simulink subsystem "MacPhersonSuspensionFront"  (R2024b)
settings: Solver=VariableStepAuto  StartTime=0.0  StopTime=10.0  RelTol=1e-3
undefined symbols (not defined in the file): PlntVehCGHgtAxl, PlntWhlNumFrnt
libraries: autolibsharedcommon x4, autolibutils x2, sharedtransform x2, matrix_library x2, vehdynlibsuspension x1
settings Model: ModifiedByFormat=The MathWorks, Inc.  Creator=The MathWorks, Inc.  LastModifiedBy=The MathWorks, Inc.
settings OptimizationCC: ReuseModelBlockBuffer=off
settings DebuggingCC: SubsystemReferenceDiagnosticForUnitTest=warning
settings RTWCC: GPUComputeCapability=3.5

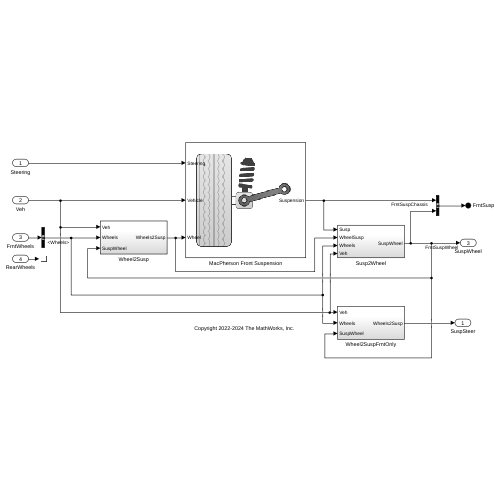
[thumbnail: Simulink's stored preview of the top-level diagram]
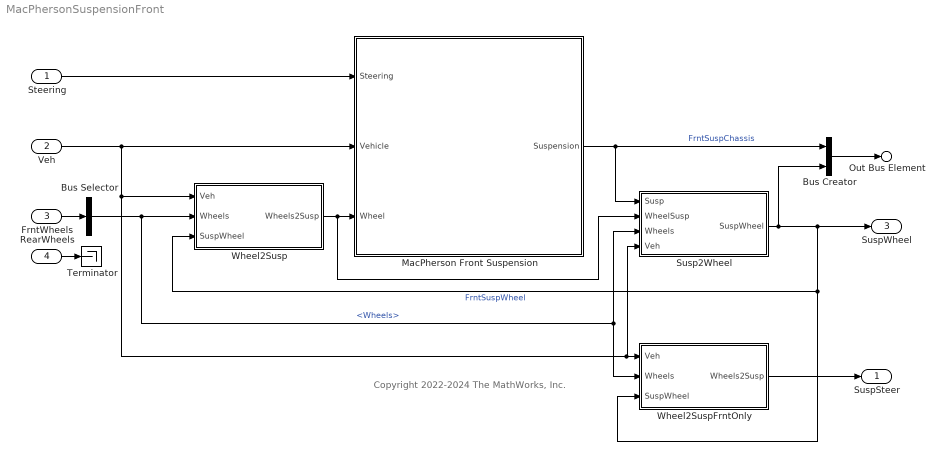
== system MacPhersonSuspensionFront ==
  note: Copyright 2022-2024 The MathWorks, Inc.
  Steering : Inport
  Veh : Inport  Port=2
  FrntWheels : Inport  Port=3
  RearWheels : Inport  Port=4
  Bus Creator : BusCreator  Inputs=2
  Bus Selector : BusSelector  OutputSignals=Wheels
  MacPherson Front Suspension : Subsystem  VariantControl=MacPherson Front Suspension Solid Axle Rear Suspension
      mask Display: image([imread('suspmacp.png')]);
  Susp2Wheel : Subsystem
  Terminator : Terminator
  Wheel2Susp : Subsystem
  Wheel2SuspFrntOnly : Subsystem
  SuspSteer : Outport
  Out Bus Element : Outport  Port=2  PortName=FrntSusp
  SuspWheel : Outport  Port=3
  wires:
  Veh/1 -> MacPherson Front Suspension/2(Vehicle), Susp2Wheel/4(Veh), Wheel2SuspFrntOnly/1(Veh), Wheel2Susp/1(Veh)
  Susp2Wheel/1(SuspWheel) -> Bus Creator/2, Wheel2SuspFrntOnly/3(SuspWheel), Wheel2Susp/3(SuspWheel), SuspWheel/1  "FrntSuspWheel"
  MacPherson Front Suspension/1(Suspension) -> Susp2Wheel/1(Susp), Bus Creator/1  "FrntSuspChassis"
  Wheel2Susp/1(Wheels2Susp) -> MacPherson Front Suspension/3(Wheel), Susp2Wheel/2(WheelSusp)
  Steering/1 -> MacPherson Front Suspension/1(Steering)
  Bus Selector/1 -> Susp2Wheel/3(Wheels), Wheel2SuspFrntOnly/2(Wheels), Wheel2Susp/2(Wheels)  "<Wheels>"
  RearWheels/1 -> Terminator/1
  FrntWheels/1 -> Bus Selector/1
  Bus Creator/1 -> Out Bus Element/1
  Wheel2SuspFrntOnly/1(Wheels2Susp) -> SuspSteer/1

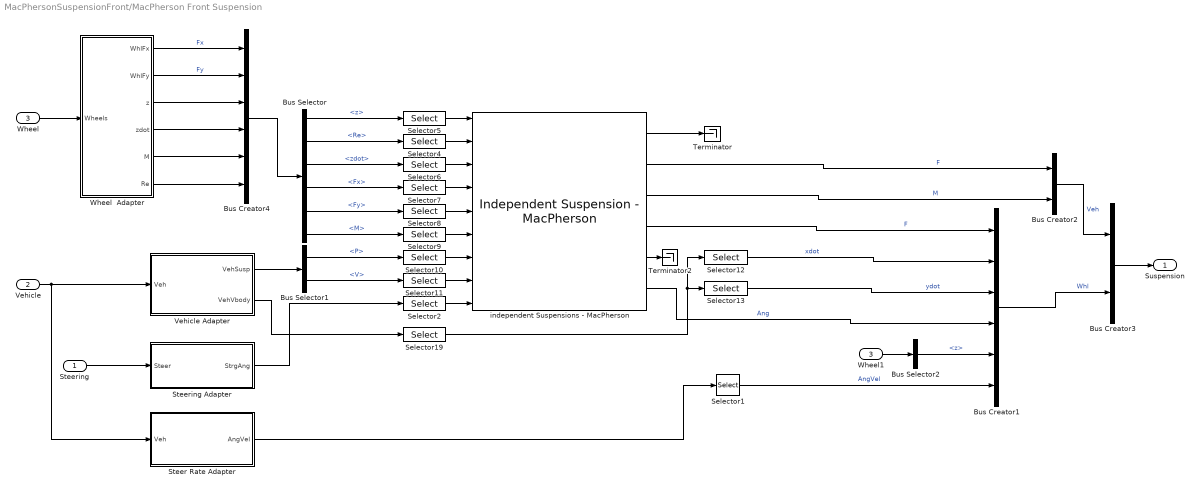
== system MacPhersonSuspensionFront/MacPherson Front Suspension ==
  Steering : Inport
  Vehicle : Inport  Port=2
  Wheel : Inport  Port=3
  Bus Creator1 : BusCreator  Inputs=6
  Bus Creator2 : BusCreator  Inputs=2
  Bus Creator3 : BusCreator  Inputs=2
  Bus Creator4 : BusCreator  Inputs=6
  Bus Selector : BusSelector  OutputSignals=z,Re,zdot,Fx,Fy,M
  Bus Selector1 : BusSelector  OutputSignals=P,V
  Bus Selector2 : BusSelector  OutputSignals=SuspFrame.z
  Selector1 : Selector  NumberOfDimensions=2  InputPortWidth=4  IndexOptions=Index vector (dialog),Index vector (dialog)  Indices=[1 2 3],[1 2]  OutputSizes=1,1
  Selector{9..11,19} (4 alike) : Selector  NumberOfDimensions=2  IndexOptions=Select all,Index vector (dialog)  Indices=[1 2],[1 2]  OutputSizes=1,1
  Selector12 : Selector  NumberOfDimensions=2  InputPortWidth=3  IndexOptions=Index vector (dialog),Select all  Indices=1,1  OutputSizes=1,1
  Selector13 : Selector  NumberOfDimensions=2  InputPortWidth=3  IndexOptions=Index vector (dialog),Select all  Indices=2,1  OutputSizes=1,1
  Selector{2,4..8} (6 alike) : Selector  IndexOptions=Index vector (dialog)  Indices=[1 2]  OutputSizes=1
  Steer Rate Adapter : Subsystem
  Steering Adapter : Subsystem
  Terminator : Terminator
  Terminator2 : Terminator
  Vehicle Adapter : Subsystem
  Wheel  Adapter : Subsystem
  Wheel1 : InportShadow  Port=3
  independent Suspensions - MacPherson : vehdynlibsuspension/Independent Suspension - MacPherson  ActiveDampEn=off  NumAxl=1  NumWhlsByAxl=2  StrgEnByAxl=1  AntiSwayEnByAxl=1  WhlNumVec="[1  2]"  AxleNumVec="[1  1]"  SuspTypesByAxle=[1]  SuspImage=suspmacp.png  IdealSuspEn=on  IdealSuspAxles=[1]  Kz=PlntSpMSStiffness  F0z=PlntSpMSPreload  Cz=PlntSpMSDamping  Hmax=PlntSpMSMaxHeight  f_act_susp_cz=[10000 10000;10000 10000]  f_act_susp_duty_bpt=[0 1]  f_act_susp_zdot_bpt=[-1 1]  Toe=PlntSpMSStatToe  RollStrgSlp=0.  ToeStrgSlp=0.  Caster=PlntSpMSStatCaster  CasterHslp=0.  CasterStrgSlp=0.  Camber=PlntSpMSStatCamber  CamberHslp=0.  CamberStrgSlp=0.  StrgHgtSlp=PlntSpMSHeightVsSteer  MappedSuspEn=off  MappedSuspAxles="[1  2]"  f_susp_axl_bp=[1 2]  f_susp_dz_bp=[-0.15 -0.14 -0.13 -0.12 -0.11 -0.10 -0.09 -0.08 -0.07 -0.06 -0.05 -0.04 -0.03 -0.02 -0.01 0.00 0.01 0.02 0.03 0.04 0.05 0.06 0.07 0.08 0.09 0.10 0.11 0.12 0.13 0.14 0.15]  f_susp_dzdot_bp=[-0.15 -0.14 -0.13 -0.12 -0.11 -0.10 -0.09 -0.08 -0.07 -0.06 -0.05 -0.04 -0.03 -0.02 -0.01 0.00 0.01 0.02 0.03 0.04 0.05 0.06 0.07 0.08 0.09 0.10 0.11 0.12 0.13 0.14 0.15]  f_susp_fmz=zeros(31,31,61,2,4)  f_susp_geom=zeros(31,61,2,3)  f_susp_strgdelta_bp=[-30,-29,-28,-27,-26,-25,-24,-23,-22,-21,-20,-19,-18,-17,-16,-15,-14,-13,-12,-11,-10,-9,-8,-7,-6,-5,-4,-3,-2,-1,0,1,2,3,4,5,6,7,8,9,10,11,12,13,14,15,16,17,18,19,20,21,22,23,24,25,26,27,28,29,30]  AntiSwayR=PlntSpMSAntiSwayRadius  AntiSwayNtrlAng=PlntSpMSAntiSwayNeutralAngle  AntiSwayTrsK=PlntSpMSAntiSwayTorsionStiffness
  Suspension : Outport  VectorParamsAs1DForOutWhenUnconnected=off
  wires:
  Selector1/1 -> Bus Creator1/6  "AngVel"
  Bus Selector2/1 -> Bus Creator1/5  "<z>"
  Wheel1/1 -> Bus Selector2/1
  Selector19/1 -> Selector13/1, Selector12/1
  independent Suspensions - MacPherson/5 -> Terminator2/1
  Steer Rate Adapter/1(AngVel) -> Selector1/1
  Vehicle Adapter/2(VehVbody) -> Selector19/1
  Bus Selector/3 -> Selector6/1  "<zdot>"
  Vehicle/1 -> Steer Rate Adapter/1(Veh), Vehicle Adapter/1(Veh)
  Wheel  Adapter/6(Re) -> Bus Creator4/6
  independent Suspensions - MacPherson/2 -> Bus Creator2/1  "F"
  independent Suspensions - MacPherson/3 -> Bus Creator2/2  "M"
  independent Suspensions - MacPherson/4 -> Bus Creator1/1  "F"
  independent Suspensions - MacPherson/6 -> Bus Creator1/4  "Ang"
  Selector12/1 -> Bus Creator1/2  "xdot"
  Selector11/1 -> independent Suspensions - MacPherson/8
  Selector10/1 -> independent Suspensions - MacPherson/7
  Selector9/1 -> independent Suspensions - MacPherson/6
  Selector8/1 -> independent Suspensions - MacPherson/5
  Selector7/1 -> independent Suspensions - MacPherson/4
  Selector6/1 -> independent Suspensions - MacPherson/3
  Selector5/1 -> independent Suspensions - MacPherson/1
  Selector4/1 -> independent Suspensions - MacPherson/2
  Selector2/1 -> independent Suspensions - MacPherson/9
  Bus Selector/2 -> Selector4/1  "<Re>"
  Wheel  Adapter/5(M) -> Bus Creator4/5
  Wheel  Adapter/4(zdot) -> Bus Creator4/4
  Wheel  Adapter/3(z) -> Bus Creator4/3
  Wheel/1 -> Wheel  Adapter/1(Wheels)
  Wheel  Adapter/1(WhlFx) -> Bus Creator4/1  "Fx"
  Wheel  Adapter/2(WhlFy) -> Bus Creator4/2  "Fy"
  Bus Creator4/1 -> Bus Selector/1
  Steering Adapter/1(StrgAng) -> Selector2/1
  Bus Creator2/1 -> Bus Creator3/1  "Veh"
  Vehicle Adapter/1(VehSusp) -> Bus Selector1/1
  Bus Selector/4 -> Selector7/1  "<Fx>"
  independent Suspensions - MacPherson/1 -> Terminator/1
  Selector13/1 -> Bus Creator1/3  "ydot"
  Bus Selector1/1 -> Selector10/1  "<P>"
  Steering/1 -> Steering Adapter/1(Steer)
  Bus Selector/1 -> Selector5/1  "<z>"
  Bus Selector/5 -> Selector8/1  "<Fy>"
  Bus Selector/6 -> Selector9/1  "<M>"
  Bus Selector1/2 -> Selector11/1  "<V>"
  Bus Creator1/1 -> Bus Creator3/2  "Whl"
  Bus Creator3/1 -> Suspension/1

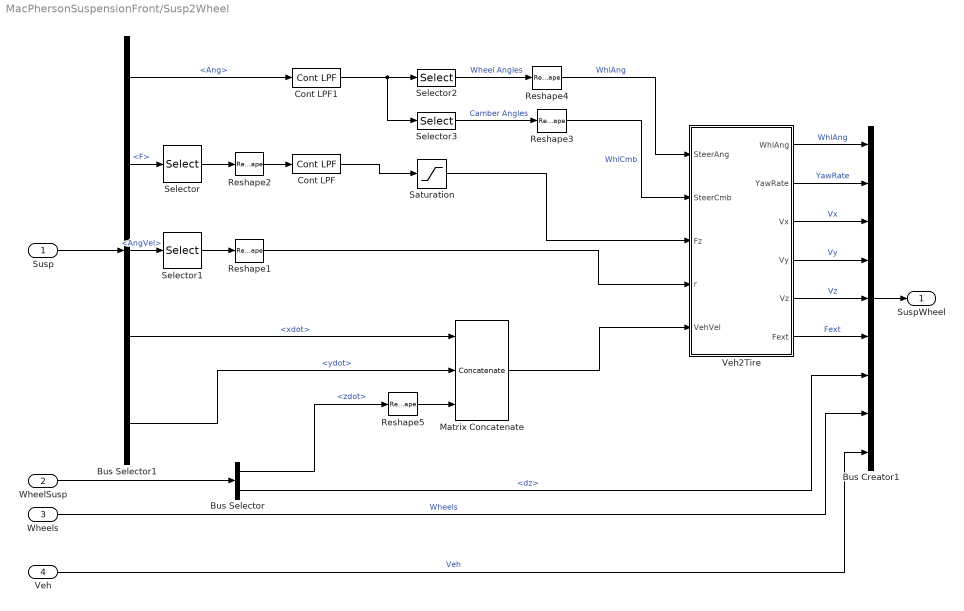
== system MacPhersonSuspensionFront/Susp2Wheel ==
  Susp : Inport
  WheelSusp : Inport  Port=2
  Wheels : Inport  Port=3
  Veh : Inport  Port=4
  Bus Creator1 : BusCreator  Inputs=9
  Bus Selector : BusSelector  OutputSignals=SuspFrame.zdot,SuspFrame.dz
  Bus Selector1 : BusSelector  OutputSignals=Whl.Ang,Whl.F,Whl.AngVel,Whl.xdot,Whl.ydot
  Cont LPF : autolibutils/Cont LPF  wc=100*2*pi  AbsoluteTolerance=auto  aMode=2
  Cont LPF1 : autolibutils/Cont LPF  wc=100*2*pi  AbsoluteTolerance=auto  aMode=2
  Matrix Concatenate : Concatenate  NumInputs=3  Mode=Multidimensional array
  Reshape{1..4} (4 alike) : Reshape
  Reshape5 : Reshape  OutputDimensionality=Row vector (2-D)
  Saturation : Saturate  UpperLimit=inf  LowerLimit=-10*9.81*2000  ZeroCross=off
  Selector : Selector  NumberOfDimensions=2  InputPortWidth=3  IndexOptions=Index vector (dialog),Select all  Indices=[3],1  OutputSizes=1,1
  Selector1 : Selector  NumberOfDimensions=2  InputPortWidth=1  IndexOptions=Index vector (dialog),Select all  Indices=[3],1  OutputSizes=1,1
  Selector2 : Selector  NumberOfDimensions=2  InputPortWidth=3  IndexOptions=Index vector (dialog),Select all  Indices=3,1  OutputSizes=1,1
  Selector3 : Selector  NumberOfDimensions=2  InputPortWidth=3  IndexOptions=Index vector (dialog),Select all  Indices=1,1  OutputSizes=1,1
  Veh2Tire : Subsystem
  SuspWheel : Outport
  wires:
  Bus Creator1/1 -> SuspWheel/1
  Bus Selector/1 -> Reshape5/1  "<zdot>"
  Veh2Tire/3(Vx) -> Bus Creator1/3  "Vx"
  Veh2Tire/4(Vy) -> Bus Creator1/4  "Vy"
  Susp/1 -> Bus Selector1/1
  Veh2Tire/5(Vz) -> Bus Creator1/5  "Vz"
  Bus Selector1/1 -> Cont LPF1/1  "<Ang>"
  Reshape5/1 -> Matrix Concatenate/3
  WheelSusp/1 -> Bus Selector/1
  Cont LPF/1 -> Saturation/1
  Selector/1 -> Reshape2/1
  Matrix Concatenate/1 -> Veh2Tire/5(VehVel)
  Saturation/1 -> Veh2Tire/3(Fz)
  Selector1/1 -> Reshape1/1
  Veh2Tire/6(Fext) -> Bus Creator1/6  "Fext"
  Bus Selector1/5 -> Matrix Concatenate/2  "<ydot>"
  Bus Selector1/3 -> Selector1/1  "<AngVel>"
  Bus Selector1/4 -> Matrix Concatenate/1  "<xdot>"
  Reshape4/1 -> Veh2Tire/1(SteerAng)  "WhlAng"
  Veh2Tire/1(WhlAng) -> Bus Creator1/1  "WhlAng"
  Reshape3/1 -> Veh2Tire/2(SteerCmb)  "WhlCmb"
  Selector3/1 -> Reshape3/1  "Camber Angles"
  Reshape2/1 -> Cont LPF/1
  Selector2/1 -> Reshape4/1  "Wheel Angles"
  Reshape1/1 -> Veh2Tire/4(r)
  Cont LPF1/1 -> Selector3/1, Selector2/1
  Bus Selector1/2 -> Selector/1  "<F>"
  Veh2Tire/2(YawRate) -> Bus Creator1/2  "YawRate"
  Bus Selector/2 -> Bus Creator1/7  "<dz>"
  Wheels/1 -> Bus Creator1/8  "Wheels"
  Veh/1 -> Bus Creator1/9  "Veh"

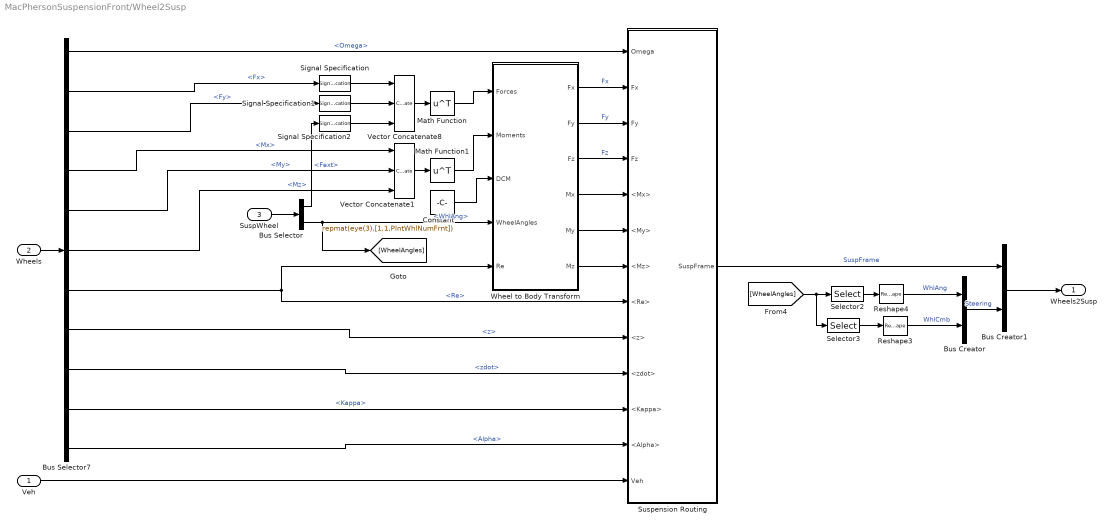
== system MacPhersonSuspensionFront/Wheel2Susp ==
  Veh : Inport
  Wheels : Inport  Port=2
  SuspWheel : Inport  Port=3
  Bus Creator : BusCreator  Inputs=2
  Bus Creator1 : BusCreator  Inputs=2
  Bus Selector : BusSelector  OutputSignals=Fext,WhlAng
  Bus Selector7 : BusSelector  OutputSignals=Omega,Fx,Fy,Mx,My,Mz,Re,z,zdot,Kappa,Alpha
  Constant : Constant  Value=repmat(eye(3),[1,1,PlntWhlNumFrnt])
  Math Function : Math  Operator=transpose  SignedPower=on
  Math Function1 : Math  Operator=transpose  SignedPower=on
  Reshape3 : Reshape
  Reshape4 : Reshape
  Selector2 : Selector  NumberOfDimensions=2  InputPortWidth=3  IndexOptions=Index vector (dialog),Select all  Indices=3,1  OutputSizes=1,1
  Selector3 : Selector  NumberOfDimensions=2  InputPortWidth=3  IndexOptions=Index vector (dialog),Select all  Indices=1,1  OutputSizes=1,1
  Signal Specification : SignalSpecification  Dimensions=PlntWhlNumFrnt
  Signal Specification1 : SignalSpecification  Dimensions=PlntWhlNumFrnt
  Signal Specification2 : SignalSpecification  Dimensions=PlntWhlNumFrnt
  Suspension Routing : Subsystem
  Vector Concatenate1 : Concatenate  NumInputs=3  Mode=Multidimensional array  ConcatenateDimension=2
  Vector Concatenate8 : Concatenate  NumInputs=3  Mode=Multidimensional array  ConcatenateDimension=2
  Wheel to Body Transform : Subsystem
  Wheels2Susp : Outport  VectorParamsAs1DForOutWhenUnconnected=off
  wires:
  Bus Selector7/11 -> Suspension Routing/12(<Alpha>)  "<Alpha>"
  Bus Selector7/10 -> Suspension Routing/11(<Kappa>)  "<Kappa>"
  Bus Selector7/9 -> Suspension Routing/10(<zdot>)  "<zdot>"
  Bus Selector7/8 -> Suspension Routing/9(<z>)  "<z>"
  Bus Selector7/7 -> Suspension Routing/8(<Re>), Wheel to Body Transform/5(Re)  "<Re>"
  Bus Selector7/6 -> Vector Concatenate1/3  "<Mz>"
  Bus Selector7/5 -> Vector Concatenate1/2  "<My>"
  Bus Selector7/4 -> Vector Concatenate1/1  "<Mx>"
  Bus Selector7/3 -> Signal Specification1/1  "<Fy>"
  Bus Selector7/2 -> Signal Specification/1  "<Fx>"
  Bus Selector7/1 -> Suspension Routing/1(Omega)  "<Omega>"
  Constant/1 -> Wheel to Body Transform/3(DCM)
  Math Function1/1 -> Wheel to Body Transform/2(Moments)
  Vector Concatenate1/1 -> Math Function1/1
  Wheel to Body Transform/6(Mz) -> Suspension Routing/7(<Mz>)
  Wheel to Body Transform/5(My) -> Suspension Routing/6(<My>)
  Wheel to Body Transform/4(Mx) -> Suspension Routing/5(<Mx>)
  Selector3/1 -> Reshape3/1
  [WheelAngles] -> Selector3/1, Selector2/1
  Selector2/1 -> Reshape4/1
  Signal Specification2/1 -> Vector Concatenate8/3
  Bus Selector/1 -> Signal Specification2/1  "<Fext>"
  SuspWheel/1 -> Bus Selector/1
  Wheel to Body Transform/2(Fy) -> Suspension Routing/3(Fy)  "Fy"
  Wheel to Body Transform/1(Fx) -> Suspension Routing/2(Fx)  "Fx"
  Vector Concatenate8/1 -> Math Function/1
  Math Function/1 -> Wheel to Body Transform/1(Forces)
  Wheels/1 -> Bus Selector7/1
  Bus Selector/2 -> Wheel to Body Transform/4(WheelAngles), [WheelAngles]  "<WhlAng>"
  Wheel to Body Transform/3(Fz) -> Suspension Routing/4(Fz)  "Fz"
  Reshape4/1 -> Bus Creator/1  "WhlAng"
  Bus Creator1/1 -> Wheels2Susp/1
  Suspension Routing/1(SuspFrame) -> Bus Creator1/1  "SuspFrame"
  Reshape3/1 -> Bus Creator/2  "WhlCmb"
  Bus Creator/1 -> Bus Creator1/2  "Steering"
  Veh/1 -> Suspension Routing/13(Veh)
  Signal Specification/1 -> Vector Concatenate8/1
  Signal Specification1/1 -> Vector Concatenate8/2

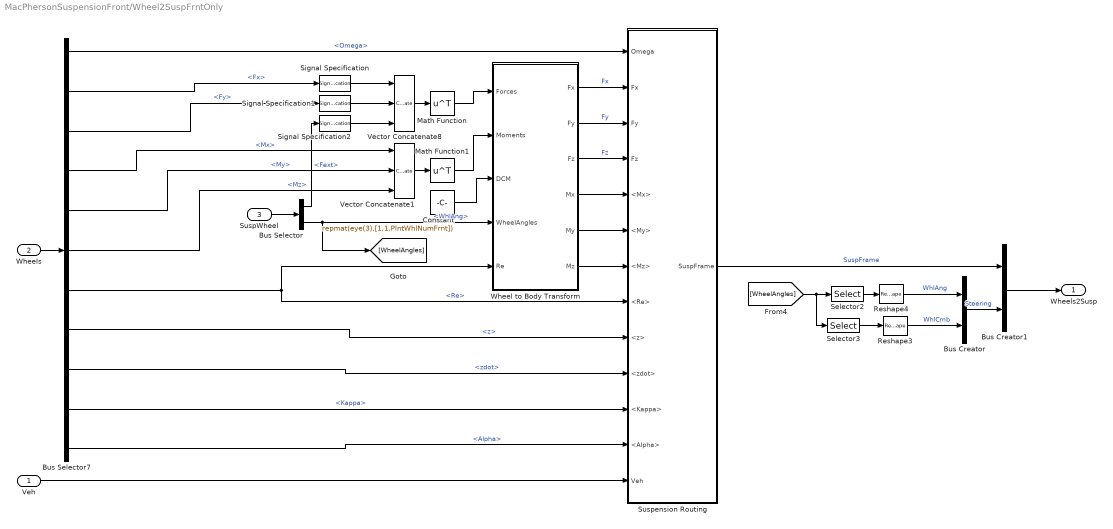
== system MacPhersonSuspensionFront/Wheel2SuspFrntOnly ==
  Veh : Inport
  Wheels : Inport  Port=2
  SuspWheel : Inport  Port=3
  Bus Creator : BusCreator  Inputs=2
  Bus Creator1 : BusCreator  Inputs=2
  Bus Selector : BusSelector  OutputSignals=Fext,WhlAng
  Bus Selector7 : BusSelector  OutputSignals=Omega,Fx,Fy,Mx,My,Mz,Re,z,zdot,Kappa,Alpha
  Constant : Constant  Value=repmat(eye(3),[1,1,PlntWhlNumFrnt])
  Math Function : Math  Operator=transpose  SignedPower=on
  Math Function1 : Math  Operator=transpose  SignedPower=on
  Reshape3 : Reshape
  Reshape4 : Reshape
  Selector2 : Selector  NumberOfDimensions=2  InputPortWidth=3  IndexOptions=Index vector (dialog),Select all  Indices=3,1  OutputSizes=1,1
  Selector3 : Selector  NumberOfDimensions=2  InputPortWidth=3  IndexOptions=Index vector (dialog),Select all  Indices=1,1  OutputSizes=1,1
  Signal Specification : SignalSpecification  Dimensions=PlntWhlNumFrnt
  Signal Specification1 : SignalSpecification  Dimensions=PlntWhlNumFrnt
  Signal Specification2 : SignalSpecification  Dimensions=PlntWhlNumFrnt
  Suspension Routing : Subsystem
  Vector Concatenate1 : Concatenate  NumInputs=3  Mode=Multidimensional array  ConcatenateDimension=2
  Vector Concatenate8 : Concatenate  NumInputs=3  Mode=Multidimensional array  ConcatenateDimension=2
  Wheel to Body Transform : Subsystem
  Wheels2Susp : Outport  VectorParamsAs1DForOutWhenUnconnected=off
  wires:
  Bus Selector7/11 -> Suspension Routing/12(<Alpha>)  "<Alpha>"
  Bus Selector7/10 -> Suspension Routing/11(<Kappa>)  "<Kappa>"
  Bus Selector7/9 -> Suspension Routing/10(<zdot>)  "<zdot>"
  Bus Selector7/8 -> Suspension Routing/9(<z>)  "<z>"
  Bus Selector7/7 -> Suspension Routing/8(<Re>), Wheel to Body Transform/5(Re)  "<Re>"
  Bus Selector7/6 -> Vector Concatenate1/3  "<Mz>"
  Bus Selector7/5 -> Vector Concatenate1/2  "<My>"
  Bus Selector7/4 -> Vector Concatenate1/1  "<Mx>"
  Bus Selector7/3 -> Signal Specification1/1  "<Fy>"
  Bus Selector7/2 -> Signal Specification/1  "<Fx>"
  Bus Selector7/1 -> Suspension Routing/1(Omega)  "<Omega>"
  Constant/1 -> Wheel to Body Transform/3(DCM)
  Math Function1/1 -> Wheel to Body Transform/2(Moments)
  Vector Concatenate1/1 -> Math Function1/1
  Wheel to Body Transform/6(Mz) -> Suspension Routing/7(<Mz>)
  Wheel to Body Transform/5(My) -> Suspension Routing/6(<My>)
  Wheel to Body Transform/4(Mx) -> Suspension Routing/5(<Mx>)
  Selector3/1 -> Reshape3/1
  [WheelAngles] -> Selector3/1, Selector2/1
  Selector2/1 -> Reshape4/1
  Signal Specification2/1 -> Vector Concatenate8/3
  Bus Selector/1 -> Signal Specification2/1  "<Fext>"
  SuspWheel/1 -> Bus Selector/1
  Wheel to Body Transform/2(Fy) -> Suspension Routing/3(Fy)  "Fy"
  Wheel to Body Transform/1(Fx) -> Suspension Routing/2(Fx)  "Fx"
  Vector Concatenate8/1 -> Math Function/1
  Math Function/1 -> Wheel to Body Transform/1(Forces)
  Wheels/1 -> Bus Selector7/1
  Bus Selector/2 -> Wheel to Body Transform/4(WheelAngles), [WheelAngles]  "<WhlAng>"
  Wheel to Body Transform/3(Fz) -> Suspension Routing/4(Fz)  "Fz"
  Reshape4/1 -> Bus Creator/1  "WhlAng"
  Bus Creator1/1 -> Wheels2Susp/1
  Suspension Routing/1(SuspFrame) -> Bus Creator1/1  "SuspFrame"
  Reshape3/1 -> Bus Creator/2  "WhlCmb"
  Bus Creator/1 -> Bus Creator1/2  "Steering"
  Veh/1 -> Suspension Routing/13(Veh)
  Signal Specification/1 -> Vector Concatenate8/1
  Signal Specification1/1 -> Vector Concatenate8/2

== system MacPhersonSuspensionFront/MacPherson Front Suspension/Steer Rate Adapter ==
  Veh : Inport
  Add : Sum
  Bus Selector3 : BusSelector  OutputSignals=BdyFrm.Cg.AngVel.r
  Constant : Constant  Value=zeros(1,4)  SampleTime=-1
  Matrix Concatenate : Concatenate  NumInputs=3  Mode=Multidimensional array
  Matrix Concatenate1 : Concatenate  NumInputs=3  Mode=Multidimensional array
  Reshape2 : Reshape  OutputDimensionality=Row vector (2-D)
  Reshape3 : Reshape  OutputDimensionality=Row vector (2-D)
  Reshape4 : Reshape  OutputDimensionality=Row vector (2-D)
  Selector3 : Selector  InputPortWidth=1  IndexOptions=Index vector (dialog)  Indices=[1 1 1 1]  OutputSizes=1
  SteerRates : Constant  Value=zeros(1,4)  SampleTime=-1
  AngVel : Outport  VectorParamsAs1DForOutWhenUnconnected=off
  wires:
  Add/1 -> AngVel/1  "AngVel"
  Veh/1 -> Bus Selector3/1
  Matrix Concatenate1/1 -> Add/1
  Reshape3/1 -> Matrix Concatenate/1, Matrix Concatenate/2
  Reshape4/1 -> Matrix Concatenate/3
  SteerRates/1 -> Reshape2/1
  Matrix Concatenate/1 -> Add/2
  Bus Selector3/1 -> Selector3/1  "<r>"
  Selector3/1 -> Reshape4/1
  Constant/1 -> Reshape3/1
  Reshape2/1 -> Matrix Concatenate1/2, Matrix Concatenate1/3, Matrix Concatenate1/1

== system MacPhersonSuspensionFront/MacPherson Front Suspension/Steering Adapter ==
  Steer : Inport
  Reshape1 : Reshape  OutputDimensionality=Row vector (2-D)
  Selector : Selector  IndexOptions=Index vector (dialog)  Indices=[1 2]  OutputSizes=1
  StrgAng : Outport  VectorParamsAs1DForOutWhenUnconnected=off
  wires:
  Selector/1 -> Reshape1/1
  Steer/1 -> Selector/1
  Reshape1/1 -> StrgAng/1

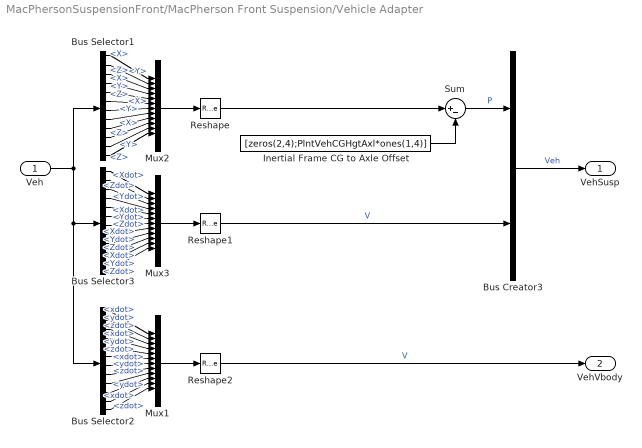
== system MacPhersonSuspensionFront/MacPherson Front Suspension/Vehicle Adapter ==
  Veh : Inport
  Bus Creator3 : BusCreator  Inputs=2
  Bus Selector1 : BusSelector  OutputSignals=InertFrm.FrntAxl.Lft.Disp.X,InertFrm.FrntAxl.Lft.Disp.Y,InertFrm.FrntAxl.Lft.Disp.Z,InertFrm.FrntAxl.Rght.Disp.X,InertFrm.FrntAxl.Rght.Disp.Y,InertFrm.FrntAxl.Rght.Disp.Z,InertFrm.RearAxl.Lft.Disp.X,InertFrm.RearAxl.Lft.Disp.Y,InertFrm.RearAxl.Lft.Disp.Z,InertFrm.RearAxl.Rght.Disp.X,InertFrm.RearAxl.Rght.Disp.Y,InertFrm.RearAxl.Rght.Disp.Z
  Bus Selector2 : BusSelector  OutputSignals=BdyFrm.FrntAxl.Lft.Vel.xdot,BdyFrm.FrntAxl.Lft.Vel.ydot,BdyFrm.FrntAxl.Lft.Vel.zdot,BdyFrm.FrntAxl.Rght.Vel.xdot,BdyFrm.FrntAxl.Rght.Vel.ydot,BdyFrm.FrntAxl.Rght.Vel.zdot,BdyFrm.RearAxl.Lft.Vel.xdot,BdyFrm.RearAxl.Lft.Vel.ydot,BdyFrm.RearAxl.Lft.Vel.zdot,BdyFrm.RearAxl.Rght.Vel.xdot,BdyFrm.RearAxl.Rght.Vel.ydot,BdyFrm.RearAxl.Rght.Vel.zdot
  Bus Selector3 : BusSelector  OutputSignals=InertFrm.FrntAxl.Lft.Vel.Xdot,InertFrm.FrntAxl.Lft.Vel.Ydot,InertFrm.FrntAxl.Lft.Vel.Zdot,InertFrm.FrntAxl.Rght.Vel.Xdot,InertFrm.FrntAxl.Rght.Vel.Ydot,InertFrm.FrntAxl.Rght.Vel.Zdot,InertFrm.RearAxl.Lft.Vel.Xdot,InertFrm.RearAxl.Lft.Vel.Ydot,InertFrm.RearAxl.Lft.Vel.Zdot,InertFrm.RearAxl.Rght.Vel.Xdot,InertFrm.RearAxl.Rght.Vel.Ydot,InertFrm.RearAxl.Rght.Vel.Zdot
  Inertial Frame CG to Axle Offset : Constant  Value=[zeros(2,4);PlntVehCGHgtAxl*ones(1,4)]  SampleTime=-1
  Mux1 : Mux  Inputs=12
  Mux2 : Mux  Inputs=12
  Mux3 : Mux  Inputs=12
  Reshape : Reshape  OutputDimensionality=Customize  OutputDimensions=[3,4]
  Reshape1 : Reshape  OutputDimensionality=Customize  OutputDimensions=[3,4]
  Reshape2 : Reshape  OutputDimensionality=Customize  OutputDimensions=[3,4]
  Sum : Sum  Inputs=|+-
  VehSusp : Outport  VectorParamsAs1DForOutWhenUnconnected=off
  VehVbody : Outport  Port=2  VectorParamsAs1DForOutWhenUnconnected=off
  wires:
  Reshape1/1 -> Bus Creator3/2  "V"
  Bus Selector3/1 -> Mux3/1  "<Xdot>"
  Bus Selector3/2 -> Mux3/2  "<Ydot>"
  Bus Selector3/3 -> Mux3/3  "<Zdot>"
  Bus Selector3/4 -> Mux3/4  "<Xdot>"
  Bus Selector3/5 -> Mux3/5  "<Ydot>"
  Bus Selector3/6 -> Mux3/6  "<Zdot>"
  Bus Selector3/7 -> Mux3/7  "<Xdot>"
  Bus Selector3/8 -> Mux3/8  "<Ydot>"
  Bus Selector3/9 -> Mux3/9  "<Zdot>"
  Bus Selector3/10 -> Mux3/10  "<Xdot>"
  Bus Selector3/11 -> Mux3/11  "<Ydot>"
  Bus Selector3/12 -> Mux3/12  "<Zdot>"
  Mux3/1 -> Reshape1/1
  Sum/1 -> Bus Creator3/1  "P"
  Inertial Frame CG to Axle Offset/1 -> Sum/2
  Mux2/1 -> Reshape/1
  Mux1/1 -> Reshape2/1
  Bus Selector2/12 -> Mux1/12  "<zdot>"
  Bus Selector2/11 -> Mux1/11  "<ydot>"
  Bus Selector2/10 -> Mux1/10  "<xdot>"
  Bus Selector2/9 -> Mux1/9  "<zdot>"
  Bus Selector2/8 -> Mux1/8  "<ydot>"
  Bus Selector2/7 -> Mux1/7  "<xdot>"
  Bus Selector2/6 -> Mux1/6  "<zdot>"
  Bus Selector2/5 -> Mux1/5  "<ydot>"
  Bus Selector2/4 -> Mux1/4  "<xdot>"
  Bus Selector2/3 -> Mux1/3  "<zdot>"
  Bus Selector2/2 -> Mux1/2  "<ydot>"
  Bus Selector2/1 -> Mux1/1  "<xdot>"
  Bus Selector1/12 -> Mux2/12  "<Z>"
  Bus Selector1/11 -> Mux2/11  "<Y>"
  Bus Selector1/10 -> Mux2/10  "<X>"
  Bus Selector1/9 -> Mux2/9  "<Z>"
  Bus Selector1/8 -> Mux2/8  "<Y>"
  Bus Selector1/7 -> Mux2/7  "<X>"
  Bus Selector1/6 -> Mux2/6  "<Z>"
  Bus Selector1/5 -> Mux2/5  "<Y>"
  Bus Selector1/4 -> Mux2/4  "<X>"
  Bus Selector1/3 -> Mux2/3  "<Z>"
  Bus Selector1/2 -> Mux2/2  "<Y>"
  Bus Selector1/1 -> Mux2/1  "<X>"
  Reshape/1 -> Sum/1
  Bus Creator3/1 -> VehSusp/1  "Veh"
  Reshape2/1 -> VehVbody/1  "V"
  Veh/1 -> Bus Selector1/1, Bus Selector2/1, Bus Selector3/1

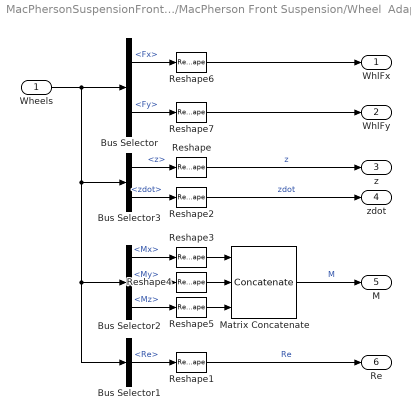
== system MacPhersonSuspensionFront/MacPherson Front Suspension/Wheel  Adapter ==
  Wheels : Inport
  Bus Selector : BusSelector  OutputSignals=SuspFrame.Fx,SuspFrame.Fy
  Bus Selector1 : BusSelector  OutputSignals=SuspFrame.Re
  Bus Selector2 : BusSelector  OutputSignals=SuspFrame.Mx,SuspFrame.My,SuspFrame.Mz
  Bus Selector3 : BusSelector  OutputSignals=SuspFrame.z,SuspFrame.zdot
  Matrix Concatenate : Concatenate  NumInputs=3  Mode=Multidimensional array
  Reshape{,1..7} (8 alike) : Reshape  OutputDimensionality=Row vector (2-D)
  WhlFx : Outport  VectorParamsAs1DForOutWhenUnconnected=off
  WhlFy : Outport  Port=2  VectorParamsAs1DForOutWhenUnconnected=off
  z : Outport  Port=3  VectorParamsAs1DForOutWhenUnconnected=off
  zdot : Outport  Port=4  VectorParamsAs1DForOutWhenUnconnected=off
  M : Outport  Port=5  VectorParamsAs1DForOutWhenUnconnected=off
  Re : Outport  Port=6  VectorParamsAs1DForOutWhenUnconnected=off
  wires:
  Reshape/1 -> z/1  "z"
  Matrix Concatenate/1 -> M/1  "M"
  Reshape5/1 -> Matrix Concatenate/3
  Reshape4/1 -> Matrix Concatenate/2
  Reshape3/1 -> Matrix Concatenate/1
  Bus Selector2/3 -> Reshape5/1  "<Mz>"
  Bus Selector2/2 -> Reshape4/1  "<My>"
  Bus Selector2/1 -> Reshape3/1  "<Mx>"
  Reshape1/1 -> Re/1  "Re"
  Bus Selector1/1 -> Reshape1/1  "<Re>"
  Reshape2/1 -> zdot/1  "zdot"
  Bus Selector3/2 -> Reshape2/1  "<zdot>"
  Wheels/1 -> Bus Selector/1, Bus Selector3/1, Bus Selector2/1, Bus Selector1/1
  Bus Selector3/1 -> Reshape/1  "<z>"
  Bus Selector/2 -> Reshape7/1  "<Fy>"
  Bus Selector/1 -> Reshape6/1  "<Fx>"
  Reshape6/1 -> WhlFx/1
  Reshape7/1 -> WhlFy/1

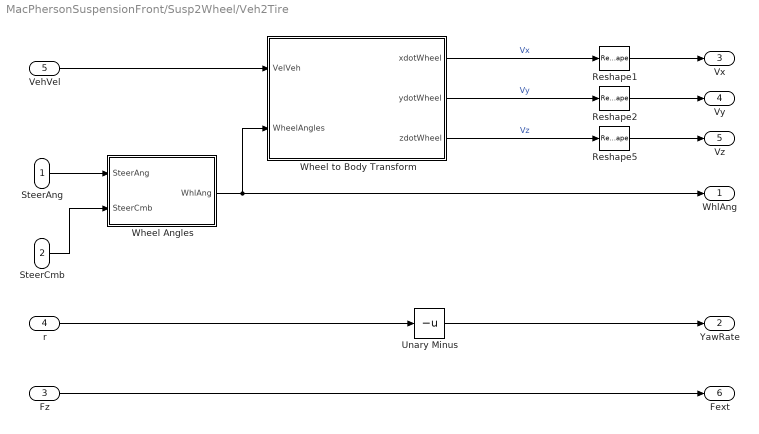
== system MacPhersonSuspensionFront/Susp2Wheel/Veh2Tire ==
  SteerAng : Inport
  SteerCmb : Inport  Port=2
  Fz : Inport  Port=3
  r : Inport  Port=4
  VehVel : Inport  Port=5
  Reshape1 : Reshape
  Reshape2 : Reshape
  Reshape5 : Reshape
  Unary Minus : UnaryMinus
  Wheel Angles : Subsystem
  Wheel to Body Transform : Subsystem
  WhlAng : Outport  Unit=rad  VectorParamsAs1DForOutWhenUnconnected=off
  YawRate : Outport  Port=2  Unit=rad/s  VectorParamsAs1DForOutWhenUnconnected=off
  Vx : Outport  Port=3  Unit=m/s  VectorParamsAs1DForOutWhenUnconnected=off
  Vy : Outport  Port=4  Unit=m/s  VectorParamsAs1DForOutWhenUnconnected=off
  Vz : Outport  Port=5  Unit=m/s  VectorParamsAs1DForOutWhenUnconnected=off
  Fext : Outport  Port=6  Unit=N  VectorParamsAs1DForOutWhenUnconnected=off
  wires:
  Fz/1 -> Fext/1
  Wheel to Body Transform/1(xdotWheel) -> Reshape1/1  "Vx"
  Wheel to Body Transform/2(ydotWheel) -> Reshape2/1  "Vy"
  SteerAng/1 -> Wheel Angles/1(SteerAng)
  r/1 -> Unary Minus/1
  VehVel/1 -> Wheel to Body Transform/1(VelVeh)
  Wheel to Body Transform/3(zdotWheel) -> Reshape5/1  "Vz"
  Unary Minus/1 -> YawRate/1
  Wheel Angles/1("WhlAng ") -> WhlAng/1, Wheel to Body Transform/2(WheelAngles)
  Reshape1/1 -> Vx/1
  Reshape2/1 -> Vy/1
  Reshape5/1 -> Vz/1
  SteerCmb/1 -> Wheel Angles/2(SteerCmb)

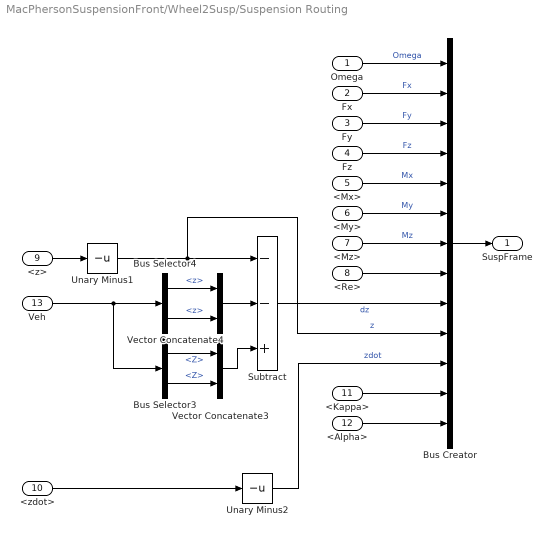
== system MacPhersonSuspensionFront/Wheel2Susp/Suspension Routing ==
  Omega : Inport
  Fx : Inport  Port=2
  Fy : Inport  Port=3
  Fz : Inport  Port=4
  <Mx> : Inport  Port=5
  <My> : Inport  Port=6
  <Mz> : Inport  Port=7
  <Re> : Inport  Port=8
  <z> : Inport  Port=9
  <zdot> : Inport  Port=10
  <Kappa> : Inport  Port=11
  <Alpha> : Inport  Port=12
  Veh : Inport  Port=13
  Bus Creator : BusCreator  Inputs=13
  Bus Selector3 : BusSelector  OutputSignals=InertFrm.FrntAxl.Lft.Disp.Z,InertFrm.FrntAxl.Rght.Disp.Z
  Bus Selector4 : BusSelector  OutputSignals=BdyFrm.FrntAxl.Lft.Disp.z,BdyFrm.FrntAxl.Rght.Disp.z
  Subtract : Sum  Inputs=--+
  Unary Minus1 : UnaryMinus
  Unary Minus2 : UnaryMinus
  Vector Concatenate3 : Concatenate
  Vector Concatenate4 : Concatenate
  SuspFrame : Outport  VectorParamsAs1DForOutWhenUnconnected=off
  wires:
  <Re>/1 -> Bus Creator/8
  Unary Minus1/1 -> Subtract/1, Bus Creator/10  "z"
  Fz/1 -> Bus Creator/4  "Fz"
  <zdot>/1 -> Unary Minus2/1
  <Mz>/1 -> Bus Creator/7  "Mz"
  Unary Minus2/1 -> Bus Creator/11  "zdot"
  <z>/1 -> Unary Minus1/1
  Bus Creator/1 -> SuspFrame/1
  Fy/1 -> Bus Creator/3  "Fy"
  Omega/1 -> Bus Creator/1  "Omega"
  Fx/1 -> Bus Creator/2  "Fx"
  <Kappa>/1 -> Bus Creator/12
  <Mx>/1 -> Bus Creator/5  "Mx"
  <My>/1 -> Bus Creator/6  "My"
  <Alpha>/1 -> Bus Creator/13
  Veh/1 -> Bus Selector3/1, Bus Selector4/1
  Subtract/1 -> Bus Creator/9  "dz"
  Bus Selector4/1 -> Vector Concatenate4/1  "<z>"
  Bus Selector3/1 -> Vector Concatenate3/1  "<Z>"
  Vector Concatenate3/1 -> Subtract/3
  Vector Concatenate4/1 -> Subtract/2
  Bus Selector4/2 -> Vector Concatenate4/2  "<z>"
  Bus Selector3/2 -> Vector Concatenate3/2  "<Z>"

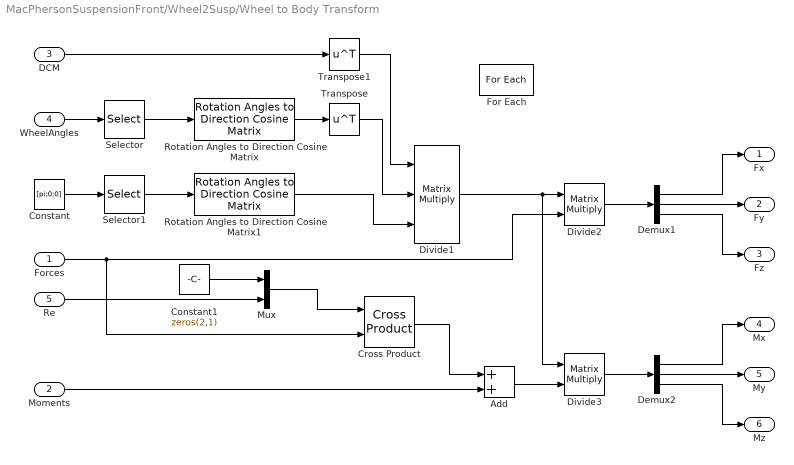
== system MacPhersonSuspensionFront/Wheel2Susp/Wheel to Body Transform ==
  Forces : Inport  PortDimensions=[3,1]  Partition=on  PartitionDimension=2  PartitionWidth=1  PartitionOffset=0
  Moments : Inport  Port=2  PortDimensions=[3,1]  Partition=on  PartitionDimension=2  PartitionWidth=1  PartitionOffset=0
  DCM : Inport  Port=3  Partition=on  PartitionDimension=3  PartitionWidth=1  PartitionOffset=0
  WheelAngles : Inport  Port=4  Partition=on  PartitionDimension=2  PartitionWidth=1  PartitionOffset=0
  Re : Inport  Port=5  Partition=on  PartitionDimension=1  PartitionWidth=1  PartitionOffset=0
  Add : Sum
  Constant : Constant  Value=[pi;0;0]
  Constant1 : Constant  Value=zeros(2,1)
  Cross Product : matrix_library/Cross Product
  Demux1 : Demux  Outputs=3
  Demux2 : Demux  Outputs=3
  Divide1 : Product  Inputs=***  Multiplication=Matrix(*)
  Divide2 : Product  Inputs=**  Multiplication=Matrix(*)
  Divide3 : Product  Inputs=**  Multiplication=Matrix(*)
  For Each : ForEach  DisableCoverage=on
  Mux : Mux  Inputs=2
  Rotation Angles to Direction Cosine Matrix : autolibsharedcommon/Rotation Angles to Direction Cosine Matrix  rotationOrder=ZYX  aMode=aMode
      settings: AttributesFormatString=Rotation Order: %<rotationOrder>
  Rotation Angles to Direction Cosine Matrix1 : autolibsharedcommon/Rotation Angles to Direction Cosine Matrix  rotationOrder=ZYX  aMode=aMode
      settings: AttributesFormatString=Rotation Order: %<rotationOrder>
  Selector : Selector  InputPortWidth=3  IndexOptions=Index vector (dialog)  Indices=[3 2 1]  OutputSizes=1
  Selector1 : Selector  InputPortWidth=3  IndexOptions=Index vector (dialog)  Indices=[3 2 1]  OutputSizes=1
  Transpose : Math  Operator=transpose
  Transpose1 : Math  Operator=transpose
  Fx : Outport  ConcatenationDimension=1  VectorParamsAs1DForOutWhenUnconnected=off
  Fy : Outport  Port=2  ConcatenationDimension=1  VectorParamsAs1DForOutWhenUnconnected=off
  Fz : Outport  Port=3  ConcatenationDimension=1  VectorParamsAs1DForOutWhenUnconnected=off
  Mx : Outport  Port=4  ConcatenationDimension=1  VectorParamsAs1DForOutWhenUnconnected=off
  My : Outport  Port=5  ConcatenationDimension=1  VectorParamsAs1DForOutWhenUnconnected=off
  Mz : Outport  Port=6  ConcatenationDimension=1  VectorParamsAs1DForOutWhenUnconnected=off
  wires:
  Constant1/1 -> Mux/1
  Re/1 -> Mux/2
  Mux/1 -> Cross Product/1
  Cross Product/1 -> Add/1
  Add/1 -> Divide3/2
  Demux2/1 -> Mx/1
  Demux2/2 -> My/1
  Demux2/3 -> Mz/1
  Moments/1 -> Add/2
  Divide1/1 -> Divide2/1, Divide3/1
  Divide3/1 -> Demux2/1
  Divide2/1 -> Demux1/1
  Transpose1/1 -> Divide1/1
  DCM/1 -> Transpose1/1
  Transpose/1 -> Divide1/2
  Constant/1 -> Selector1/1
  Selector1/1 -> Rotation Angles to Direction Cosine Matrix1/1
  Rotation Angles to Direction Cosine Matrix1/1 -> Divide1/3
  Selector/1 -> Rotation Angles to Direction Cosine Matrix/1
  WheelAngles/1 -> Selector/1
  Forces/1 -> Cross Product/2, Divide2/2
  Rotation Angles to Direction Cosine Matrix/1 -> Transpose/1
  Demux1/3 -> Fz/1
  Demux1/2 -> Fy/1
  Demux1/1 -> Fx/1

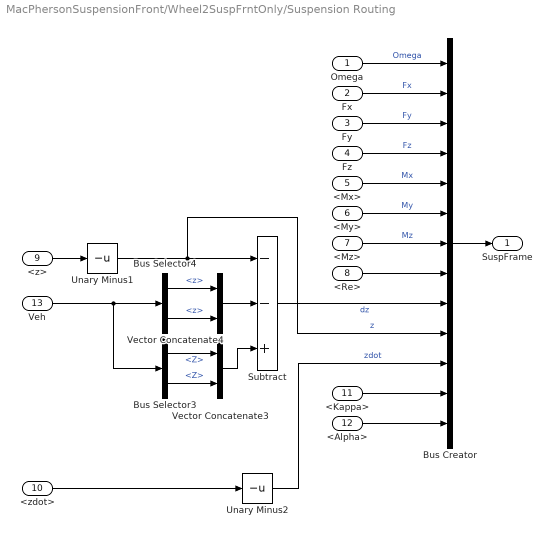
== system MacPhersonSuspensionFront/Wheel2SuspFrntOnly/Suspension Routing ==
  Omega : Inport
  Fx : Inport  Port=2
  Fy : Inport  Port=3
  Fz : Inport  Port=4
  <Mx> : Inport  Port=5
  <My> : Inport  Port=6
  <Mz> : Inport  Port=7
  <Re> : Inport  Port=8
  <z> : Inport  Port=9
  <zdot> : Inport  Port=10
  <Kappa> : Inport  Port=11
  <Alpha> : Inport  Port=12
  Veh : Inport  Port=13
  Bus Creator : BusCreator  Inputs=13
  Bus Selector3 : BusSelector  OutputSignals=InertFrm.FrntAxl.Lft.Disp.Z,InertFrm.FrntAxl.Rght.Disp.Z
  Bus Selector4 : BusSelector  OutputSignals=BdyFrm.FrntAxl.Lft.Disp.z,BdyFrm.FrntAxl.Rght.Disp.z
  Subtract : Sum  Inputs=--+
  Unary Minus1 : UnaryMinus
  Unary Minus2 : UnaryMinus
  Vector Concatenate3 : Concatenate
  Vector Concatenate4 : Concatenate
  SuspFrame : Outport  VectorParamsAs1DForOutWhenUnconnected=off
  wires:
  <Re>/1 -> Bus Creator/8
  Unary Minus1/1 -> Subtract/1, Bus Creator/10  "z"
  Fz/1 -> Bus Creator/4  "Fz"
  <zdot>/1 -> Unary Minus2/1
  <Mz>/1 -> Bus Creator/7  "Mz"
  Unary Minus2/1 -> Bus Creator/11  "zdot"
  <z>/1 -> Unary Minus1/1
  Bus Creator/1 -> SuspFrame/1
  Fy/1 -> Bus Creator/3  "Fy"
  Omega/1 -> Bus Creator/1  "Omega"
  Fx/1 -> Bus Creator/2  "Fx"
  <Kappa>/1 -> Bus Creator/12
  <Mx>/1 -> Bus Creator/5  "Mx"
  <My>/1 -> Bus Creator/6  "My"
  <Alpha>/1 -> Bus Creator/13
  Veh/1 -> Bus Selector3/1, Bus Selector4/1
  Subtract/1 -> Bus Creator/9  "dz"
  Bus Selector4/1 -> Vector Concatenate4/1  "<z>"
  Bus Selector3/1 -> Vector Concatenate3/1  "<Z>"
  Vector Concatenate3/1 -> Subtract/3
  Vector Concatenate4/1 -> Subtract/2
  Bus Selector4/2 -> Vector Concatenate4/2  "<z>"
  Bus Selector3/2 -> Vector Concatenate3/2  "<Z>"

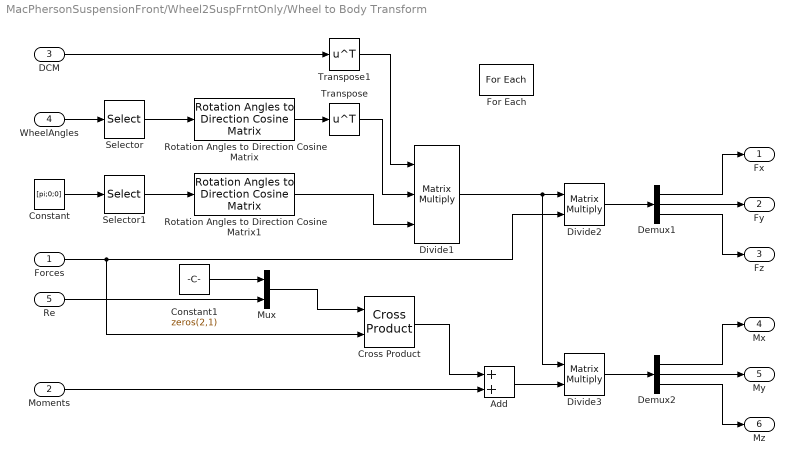
== system MacPhersonSuspensionFront/Wheel2SuspFrntOnly/Wheel to Body Transform ==
  Forces : Inport  PortDimensions=[3,1]  Partition=on  PartitionDimension=2  PartitionWidth=1  PartitionOffset=0
  Moments : Inport  Port=2  PortDimensions=[3,1]  Partition=on  PartitionDimension=2  PartitionWidth=1  PartitionOffset=0
  DCM : Inport  Port=3  Partition=on  PartitionDimension=3  PartitionWidth=1  PartitionOffset=0
  WheelAngles : Inport  Port=4  Partition=on  PartitionDimension=2  PartitionWidth=1  PartitionOffset=0
  Re : Inport  Port=5  Partition=on  PartitionDimension=1  PartitionWidth=1  PartitionOffset=0
  Add : Sum
  Constant : Constant  Value=[pi;0;0]
  Constant1 : Constant  Value=zeros(2,1)
  Cross Product : matrix_library/Cross Product
  Demux1 : Demux  Outputs=3
  Demux2 : Demux  Outputs=3
  Divide1 : Product  Inputs=***  Multiplication=Matrix(*)
  Divide2 : Product  Inputs=**  Multiplication=Matrix(*)
  Divide3 : Product  Inputs=**  Multiplication=Matrix(*)
  For Each : ForEach  DisableCoverage=on
  Mux : Mux  Inputs=2
  Rotation Angles to Direction Cosine Matrix : autolibsharedcommon/Rotation Angles to Direction Cosine Matrix  rotationOrder=ZYX  aMode=aMode
      settings: AttributesFormatString=Rotation Order: %<rotationOrder>
  Rotation Angles to Direction Cosine Matrix1 : autolibsharedcommon/Rotation Angles to Direction Cosine Matrix  rotationOrder=ZYX  aMode=aMode
      settings: AttributesFormatString=Rotation Order: %<rotationOrder>
  Selector : Selector  InputPortWidth=3  IndexOptions=Index vector (dialog)  Indices=[3 2 1]  OutputSizes=1
  Selector1 : Selector  InputPortWidth=3  IndexOptions=Index vector (dialog)  Indices=[3 2 1]  OutputSizes=1
  Transpose : Math  Operator=transpose
  Transpose1 : Math  Operator=transpose
  Fx : Outport  ConcatenationDimension=1  VectorParamsAs1DForOutWhenUnconnected=off
  Fy : Outport  Port=2  ConcatenationDimension=1  VectorParamsAs1DForOutWhenUnconnected=off
  Fz : Outport  Port=3  ConcatenationDimension=1  VectorParamsAs1DForOutWhenUnconnected=off
  Mx : Outport  Port=4  ConcatenationDimension=1  VectorParamsAs1DForOutWhenUnconnected=off
  My : Outport  Port=5  ConcatenationDimension=1  VectorParamsAs1DForOutWhenUnconnected=off
  Mz : Outport  Port=6  ConcatenationDimension=1  VectorParamsAs1DForOutWhenUnconnected=off
  wires:
  Constant1/1 -> Mux/1
  Re/1 -> Mux/2
  Mux/1 -> Cross Product/1
  Cross Product/1 -> Add/1
  Add/1 -> Divide3/2
  Demux2/1 -> Mx/1
  Demux2/2 -> My/1
  Demux2/3 -> Mz/1
  Moments/1 -> Add/2
  Divide1/1 -> Divide2/1, Divide3/1
  Divide3/1 -> Demux2/1
  Divide2/1 -> Demux1/1
  Transpose1/1 -> Divide1/1
  DCM/1 -> Transpose1/1
  Transpose/1 -> Divide1/2
  Constant/1 -> Selector1/1
  Selector1/1 -> Rotation Angles to Direction Cosine Matrix1/1
  Rotation Angles to Direction Cosine Matrix1/1 -> Divide1/3
  Selector/1 -> Rotation Angles to Direction Cosine Matrix/1
  WheelAngles/1 -> Selector/1
  Forces/1 -> Cross Product/2, Divide2/2
  Rotation Angles to Direction Cosine Matrix/1 -> Transpose/1
  Demux1/3 -> Fz/1
  Demux1/2 -> Fy/1
  Demux1/1 -> Fx/1

== system MacPhersonSuspensionFront/Susp2Wheel/Veh2Tire/Wheel Angles ==
  SteerAng : Inport
  SteerCmb : Inport  Port=2
  Constant3 : Constant  Value=ones(1,PlntWhlNumFrnt).*0  SampleTime=-1
  Reshape : Reshape  OutputDimensionality=Row vector (2-D)
  Reshape1 : Reshape  OutputDimensionality=Row vector (2-D)
  Reshape2 : Reshape  OutputDimensionality=Row vector (2-D)
  Vector Concatenate3 : Concatenate  NumInputs=3  Mode=Multidimensional array
  "WhlAng " : Outport  VectorParamsAs1DForOutWhenUnconnected=off
  wires:
  Constant3/1 -> Reshape2/1
  Vector Concatenate3/1 -> "WhlAng "/1
  Reshape/1 -> Vector Concatenate3/3
  Reshape1/1 -> Vector Concatenate3/1
  SteerCmb/1 -> Reshape1/1
  Reshape2/1 -> Vector Concatenate3/2
  SteerAng/1 -> Reshape/1

== system MacPhersonSuspensionFront/Susp2Wheel/Veh2Tire/Wheel to Body Transform ==
  VelVeh : Inport  Partition=on  PartitionDimension=2  PartitionWidth=1  PartitionOffset=0
  WheelAngles : Inport  Port=2  Partition=on  PartitionDimension=2  PartitionWidth=1  PartitionOffset=0
  Constant : Constant  Value=[pi;0;0]  SampleTime=-1
  Demux1 : Demux  Outputs=3
  Divide1 : Product  Inputs=**  Multiplication=Matrix(*)
  Divide2 : Product  Inputs=**  Multiplication=Matrix(*)
  For Each : ForEach  DisableCoverage=on
  Rotation Angles to Direction Cosine Matrix : sharedtransform/Rotation Angles to Direction Cosine Matrix  rotationOrder=ZYX  aMode=2
  Rotation Angles to Direction Cosine Matrix1 : sharedtransform/Rotation Angles to Direction Cosine Matrix  rotationOrder=ZYX  aMode=2
  Selector : Selector  InputPortWidth=3  IndexOptions=Index vector (dialog)  Indices=[3 2 1]  OutputSizes=1
  Selector1 : Selector  InputPortWidth=3  IndexOptions=Index vector (dialog)  Indices=[3 2 1]  OutputSizes=1
  xdotWheel : Outport  ConcatenationDimension=1  VectorParamsAs1DForOutWhenUnconnected=off
  ydotWheel : Outport  Port=2  ConcatenationDimension=1  VectorParamsAs1DForOutWhenUnconnected=off
  zdotWheel : Outport  Port=3  ConcatenationDimension=1  VectorParamsAs1DForOutWhenUnconnected=off
  wires:
  Divide2/1 -> Demux1/1
  Demux1/1 -> xdotWheel/1
  Demux1/2 -> ydotWheel/1
  Demux1/3 -> zdotWheel/1
  Rotation Angles to Direction Cosine Matrix/1 -> Divide1/1
  VelVeh/1 -> Divide1/2
  WheelAngles/1 -> Selector/1
  Selector/1 -> Rotation Angles to Direction Cosine Matrix/1
  Selector1/1 -> Rotation Angles to Direction Cosine Matrix1/1
  Rotation Angles to Direction Cosine Matrix1/1 -> Divide2/1
  Divide1/1 -> Divide2/2
  Constant/1 -> Selector1/1
